simulink model "Inverted_pendulum_model1"  (R2022a)
settings: Solver=VariableStepAuto  StartTime=0.0  StopTime=10  RelTol=1e-3
undefined symbols (not defined in the file): K, sys1
settings Model: Creator=tr419926  LastModifiedBy=tr419926

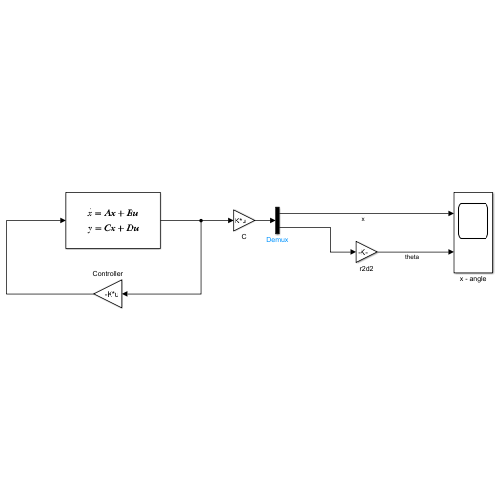
[thumbnail: Simulink's stored preview of the top-level diagram]
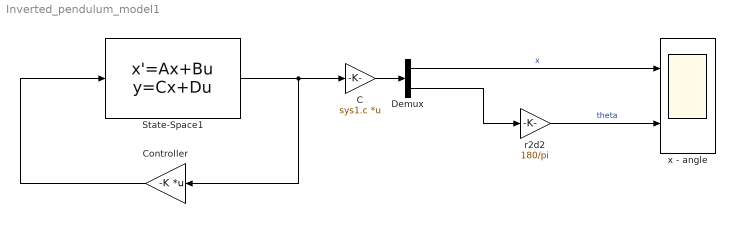
== system Inverted_pendulum_model1 ==
  C : Gain  Gain=sys1.c  Multiplication=Matrix(K*u)
  Controller : Gain  Gain=-K  Multiplication=Matrix(K*u)
  Demux : Demux  Outputs=2
  State-Space1 : StateSpace  A=sys1.a  B=sys1.b  C=eye(4)  D=zeros(4,1)  InitialCondition=[0 0 5/180*pi 0]
  r2d2 : Gain  Gain=180/pi
  x - angle : Scope  NumInputPorts=2
  wires:
  Controller/1 -> State-Space1/1
  State-Space1/1 -> C/1, Controller/1
  Demux/1 -> x - angle/1  "x"
  Demux/2 -> r2d2/1
  C/1 -> Demux/1
  r2d2/1 -> x - angle/2  "theta"
